simulink model "C1_Chirp_Filter"  (R2019b)
settings: Solver=VariableStepAuto  StartTime=0.0  StopTime=testtime  RelTol=1e-3
InitFcn:
  | C1_Chirp_Test_Parameters
StopFcn:
  | Verify_C1_Chirp_Filter
values from neighbouring files (symbols this model uses):
  C1gain_norm = C1gain_norm*((CF-pimag(i))^2 + (preal(i))^2)    [C1_Chirp_Test_Parameters.m]
  C1initphase = C1initphase + atan(CF/(-rzero))-atan((CF-pimag(2*i-1))/(-preal(2*i-1)))-atan((CF+pimag(2*i-1))/(-preal(2*i-1)))    [C1_Chirp_Test_Parameters.m]
  CF = 2*pi*cf    (= 6283.18530718)    [C1_Chirp_Test_Parameters.m]
  Fs = 48e3    (= 48000)    [C1_Chirp_Test_Parameters.m]
  fs_bilinear = 2*pi*cf/tan(2*pi*cf*tdres/2)    [C1_Chirp_Test_Parameters.m]
  norm_gainc1 = (sqrt(C1gain_norm))/((sqrt(CF^2+rzero^2))^order_of_zero)    [C1_Chirp_Test_Parameters.m]
  order_of_zero = half_order_pole    (= 5)    [C1_Chirp_Test_Parameters.m]
  pimag = zeros(11,1)    [C1_Chirp_Test_Parameters.m]
  preal = zeros(11,1)    [C1_Chirp_Test_Parameters.m]
  rsigma = 1    [C1_Chirp_Test_Parameters.m]
  rzero = -pzero    [C1_Chirp_Test_Parameters.m]
libraries: dspsrcs4 x2
settings Model: Creator=mblun  LastModifiedBy=t96f346
settings SFSimCC: CustomCodeUndefinedFunction=UseInterfaceOnly

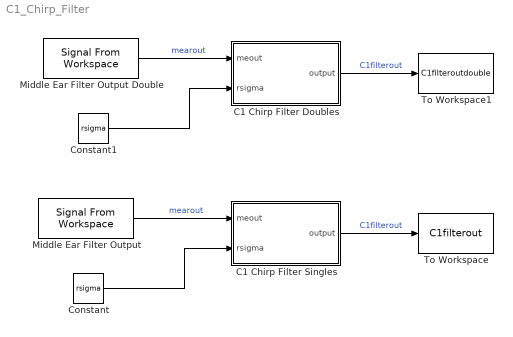
== system C1_Chirp_Filter ==
  C1 Chirp Filter Doubles : Subsystem
  C1 Chirp Filter Singles : Subsystem
  Constant : Constant  Value=rsigma  OutDataTypeStr=single  SampleTime=-1
  Constant1 : Constant  Value=rsigma  SampleTime=-1
  Middle Ear Filter Output : dspsrcs4/Signal From Workspace  X=RxSignal  Ts=1/Fs  nsamps=1  OutputAfterFinalValue=Setting to zero  ignoreOrWarnInputAndFrameLengths=off  OutputFrames=off
  Middle Ear Filter Output Double : dspsrcs4/Signal From Workspace  X=RxSignalDouble  Ts=1/Fs  nsamps=1  OutputAfterFinalValue=Setting to zero  ignoreOrWarnInputAndFrameLengths=off  OutputFrames=off
  To Workspace : ToWorkspace  VariableName=C1filterout  SampleTime=-1
      settings: Save2DSignal=2-D array (concatenate along first dimension)
  To Workspace1 : ToWorkspace  VariableName=C1filteroutdouble  SampleTime=-1
      settings: Save2DSignal=2-D array (concatenate along first dimension)
  wires:
  Middle Ear Filter Output/1 -> C1 Chirp Filter Singles/1(meout)  "mearout"
  Constant/1 -> C1 Chirp Filter Singles/2(rsigma)
  C1 Chirp Filter Singles/1(output) -> To Workspace/1  "C1filterout"
  Constant1/1 -> C1 Chirp Filter Doubles/2(rsigma)
  Middle Ear Filter Output Double/1 -> C1 Chirp Filter Doubles/1(meout)  "mearout"
  C1 Chirp Filter Doubles/1(output) -> To Workspace1/1  "C1filterout"

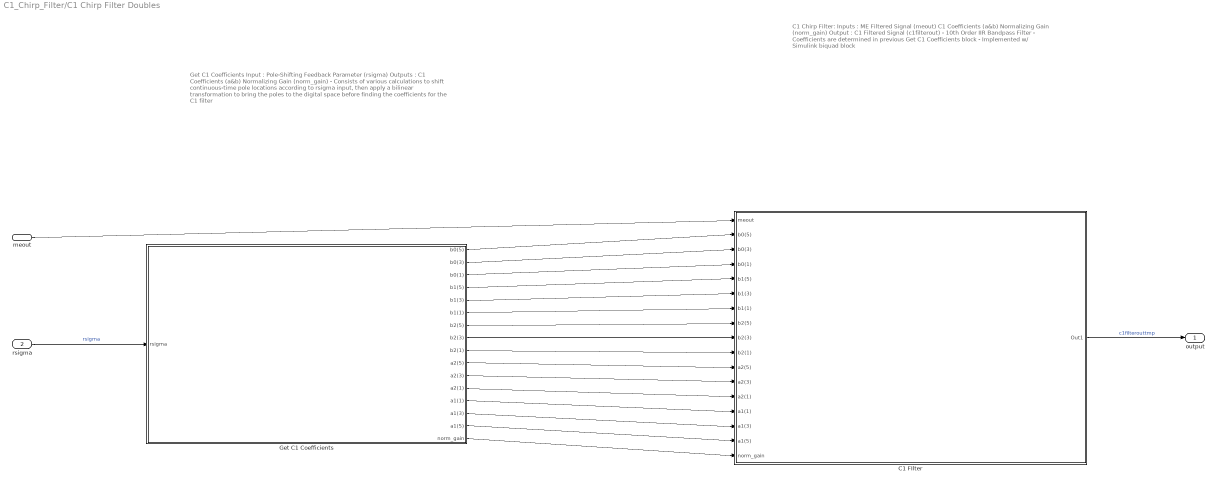
== system C1_Chirp_Filter/C1 Chirp Filter Doubles ==
  note: C1 Chirp Filter:
      |
      | Inputs : ME Filtered Signal (meout)
      | C1 Coefficients (a&b)
      | Normalizing Gain (norm_gain)
      |
      | Output : C1 Filtered Signal (c1filterout)
      |
      | - 10th Order IIR Bandpass Filter
      |
      | - Coefficients are determined in previous Get C1 Coefficients block
      |
      | - Implemented w/ Simulink biquad block
  note: Get C1 Coefficients
      |
      | Input : Pole-Shifting Feedback Parameter (rsigma)
      |
      | Outputs : C1 Coefficients (a&b)
      | Normalizing Gain (norm_gain)
      |
      | - Consists of various calculations to shift continuous-time pole locations according to rsigma input, then apply a bilinear transformation to bring the poles to the digital space before finding the coefficients for the C1 filter
  meout : Inport
  rsigma : Inport  Port=2
  C1 FIlter : Subsystem
  Get C1 Coefficients : Subsystem
  output : Outport  VectorParamsAs1DForOutWhenUnconnected=off
  wires:
  C1 FIlter/1(Out1) -> output/1  "c1filterouttmp"
  Get C1 Coefficients/1(b0(5)) -> C1 FIlter/2(b0(5))
  Get C1 Coefficients/9(b2(1)) -> C1 FIlter/10(b2(1))
  rsigma/1 -> Get C1 Coefficients/1(rsigma)  "rsigma"
  Get C1 Coefficients/10(a2(5)) -> C1 FIlter/11(a2(5))
  Get C1 Coefficients/15(a1(5)) -> C1 FIlter/16(a1(5))
  Get C1 Coefficients/6(b1(1)) -> C1 FIlter/7(b1(1))
  meout/1 -> C1 FIlter/1(meout)
  Get C1 Coefficients/16(norm_gain) -> C1 FIlter/17(norm_gain)
  Get C1 Coefficients/13(a1(1)) -> C1 FIlter/14(a1(1))
  Get C1 Coefficients/14(a1(3)) -> C1 FIlter/15(a1(3))
  Get C1 Coefficients/12(a2(1)) -> C1 FIlter/13(a2(1))
  Get C1 Coefficients/11(a2(3)) -> C1 FIlter/12(a2(3))
  Get C1 Coefficients/2(b0(3)) -> C1 FIlter/3(b0(3))
  Get C1 Coefficients/3(b0(1)) -> C1 FIlter/4(b0(1))
  Get C1 Coefficients/4(b1(5)) -> C1 FIlter/5(b1(5))
  Get C1 Coefficients/8(b2(3)) -> C1 FIlter/9(b2(3))
  Get C1 Coefficients/5(b1(3)) -> C1 FIlter/6(b1(3))
  Get C1 Coefficients/7(b2(5)) -> C1 FIlter/8(b2(5))

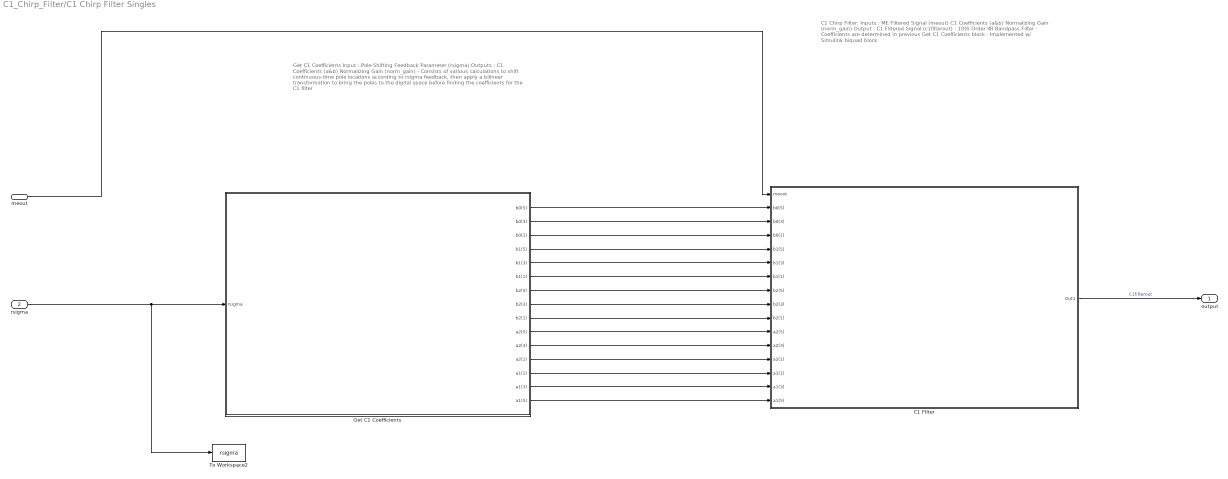
== system C1_Chirp_Filter/C1 Chirp Filter Singles ==
  note: C1 Chirp Filter:
      |
      | Inputs : ME Filtered Signal (meout)
      | C1 Coefficients (a&b)
      | Normalizing Gain (norm_gain)
      |
      | Output : C1 Filtered Signal (c1filterout)
      |
      | - 10th Order IIR Bandpass Filter
      |
      | - Coefficients are determined in previous Get C1 Coefficients block
      |
      | - Implemented w/ Simulink biquad block
  note: Get C1 Coefficients
      |
      | Input : Pole-Shifting Feedback Parameter (rsigma)
      |
      | Outputs : C1 Coefficients (a&b)
      | Normalizing Gain (norm_gain)
      |
      | - Consists of various calculations to shift continuous-time pole locations according to rsigma feedback, then apply a bilinear transformation to bring the poles to the digital space before finding the coefficients for the C1 filter
  meout : Inport
  rsigma : Inport  Port=2
  C1 FIlter : Subsystem
  Get C1 Coefficients : Subsystem
  To Workspace2 : ToWorkspace  VariableName=rsigma  SampleTime=-1
      settings: Save2DSignal=2-D array (concatenate along first dimension)
  output : Outport  VectorParamsAs1DForOutWhenUnconnected=off
  wires:
  meout/1 -> C1 FIlter/1(meout)
  Get C1 Coefficients/1(b0(5)) -> C1 FIlter/2(b0(5))
  Get C1 Coefficients/2(b0(3)) -> C1 FIlter/3(b0(3))
  Get C1 Coefficients/3(b0(1)) -> C1 FIlter/4(b0(1))
  Get C1 Coefficients/4(b1(5)) -> C1 FIlter/5(b1(5))
  Get C1 Coefficients/5(b1(3)) -> C1 FIlter/6(b1(3))
  Get C1 Coefficients/6(b1(1)) -> C1 FIlter/7(b1(1))
  Get C1 Coefficients/7(b2(5)) -> C1 FIlter/8(b2(5))
  Get C1 Coefficients/8(b2(3)) -> C1 FIlter/9(b2(3))
  Get C1 Coefficients/9(b2(1)) -> C1 FIlter/10(b2(1))
  Get C1 Coefficients/10(a2(5)) -> C1 FIlter/11(a2(5))
  Get C1 Coefficients/11(a2(3)) -> C1 FIlter/12(a2(3))
  Get C1 Coefficients/12(a2(1)) -> C1 FIlter/13(a2(1))
  Get C1 Coefficients/13(a1(1)) -> C1 FIlter/14(a1(1))
  Get C1 Coefficients/14(a1(3)) -> C1 FIlter/15(a1(3))
  Get C1 Coefficients/15(a1(5)) -> C1 FIlter/16(a1(5))
  C1 FIlter/1(Out1) -> output/1  "C1filterout"
  rsigma/1 -> To Workspace2/1, Get C1 Coefficients/1(rsigma)

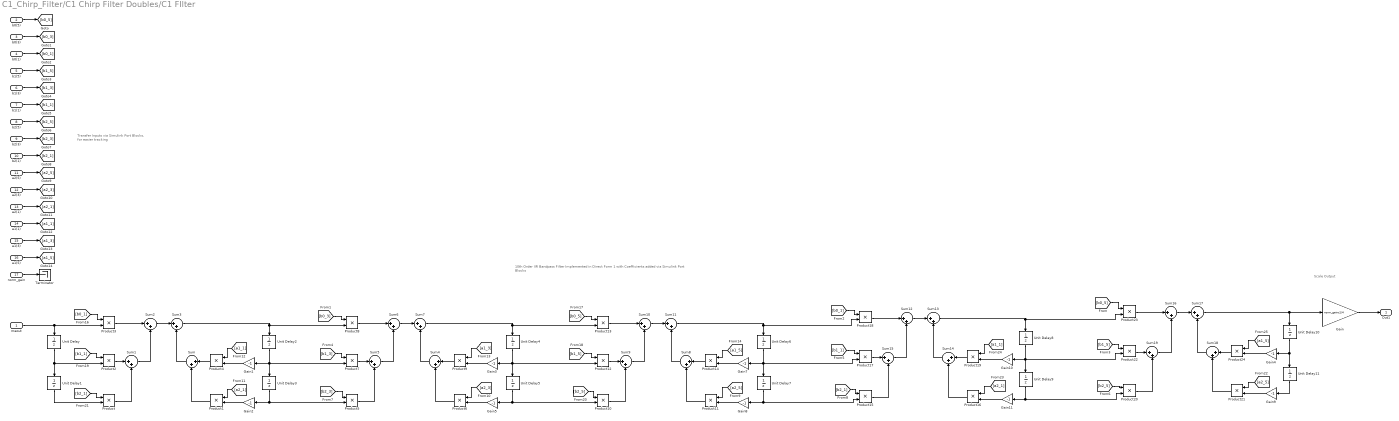
== system C1_Chirp_Filter/C1 Chirp Filter Doubles/C1 FIlter ==
  note: Transfer Inputs via Simulink Port Blocks, for easier tracking
  note: 10th Order IIR Bandpass Filter Implemented in Direct Form 1 with Coefficients added via Simulink Port Blocks
  note: Scale Output
  meout : Inport
  b0(5) : Inport  Port=2
  b0(3) : Inport  Port=3
  b0(1) : Inport  Port=4
  b1(5) : Inport  Port=5
  b1(3) : Inport  Port=6
  b1(1) : Inport  Port=7
  b2(5) : Inport  Port=8
  b2(3) : Inport  Port=9
  b2(1) : Inport  Port=10
  a2(5) : Inport  Port=11
  a2(3) : Inport  Port=12
  a2(1) : Inport  Port=13
  a1(1) : Inport  Port=14
  a1(3) : Inport  Port=15
  a1(5) : Inport  Port=16
  norm_gain : Inport  Port=17
  Gain : Gain  Gain=norm_gainc1/4
  Gain{1..5,7..11} (10 alike) : Gain  Gain=-1
  Product{,1..24} (25 alike) : Product
  Sum{,1..19} (20 alike) : Sum  Inputs=|++
  Terminator : Terminator
  Unit Delay{,1..11} (12 alike) : UnitDelay  SampleTime=-1  HasFrameUpgradeWarning=on
  Out1 : Outport  VectorParamsAs1DForOutWhenUnconnected=off
  wires:
  [a1_5] -> Product14/1
  Product15/1 -> Sum15/2
  Product16/1 -> Sum14/2
  Sum5/1 -> Sum6/2
  Sum15/1 -> Sum12/2
  Unit Delay2/1 -> Product7/2, Unit Delay3/1, Gain1/1
  Unit Delay6/1 -> Product17/2, Unit Delay7/1, Gain7/1
  [b1_3] -> Product7/1
  Sum1/1 -> Sum2/2
  [b0_1] -> Product3/1
  Product4/1 -> Sum/1
  Unit Delay8/1 -> Product22/2, Unit Delay9/1, Gain10/1
  Product12/1 -> Sum9/1
  Sum17/1 -> Unit Delay10/1, Gain/1
  Product3/1 -> Sum2/1
  [b2_3] -> Product5/1
  Sum7/1 -> Product13/2, Unit Delay4/1
  [a2_1] -> Product1/1
  [b2_1] -> Product/1
  Product24/1 -> Sum18/1
  Unit Delay3/1 -> Product5/2, Gain2/1
  Product5/1 -> Sum5/2
  Unit Delay4/1 -> Product12/2, Unit Delay5/1, Gain3/1
  Sum13/1 -> Product23/2, Unit Delay8/1
  Sum3/1 -> Product8/2, Unit Delay2/1
  Sum4/1 -> Sum7/2
  Product19/1 -> Sum14/1
  Product7/1 -> Sum5/1
  Product10/1 -> Sum9/2
  Product20/1 -> Sum19/2
  [a1_5] -> Product24/1
  Sum6/1 -> Sum7/1
  [b0_5] -> Product13/1
  [a1_3] -> Product9/1
  Product22/1 -> Sum19/1
  Product8/1 -> Sum6/1
  meout/1 -> Product3/2, Unit Delay/1
  Product2/1 -> Sum1/1
  Sum11/1 -> Product18/2, Unit Delay6/1
  Unit Delay5/1 -> Product10/2, Gain5/1
  [b1_5] -> Product12/1
  Sum2/1 -> Sum3/1
  Product11/1 -> Sum8/2
  Sum19/1 -> Sum16/2
  [b2_5] -> Product20/1
  Product14/1 -> Sum8/1
  Product18/1 -> Sum12/1
  Sum8/1 -> Sum11/2
  [b0_3] -> Product8/1
  Sum12/1 -> Sum13/1
  [b0_5] -> Product23/1
  [b0_1] -> Product18/1
  [a1_1] -> Product19/1
  [a2_5] -> Product21/1
  Unit Delay/1 -> Unit Delay1/1, Product2/2
  Product17/1 -> Sum15/1
  Unit Delay7/1 -> Product15/2, Gain8/1
  Unit Delay10/1 -> Unit Delay11/1, Gain4/1
  [a2_5] -> Product11/1
  Unit Delay11/1 -> Gain9/1
  Gain/1 -> Out1/1
  Product23/1 -> Sum16/1
  Product9/1 -> Sum4/1
  [b1_1] -> Product17/1
  Product13/1 -> Sum10/1
  Product6/1 -> Sum4/2
  Sum9/1 -> Sum10/2
  Sum16/1 -> Sum17/1
  Product21/1 -> Sum18/2
  [b1_1] -> Product2/1
  Sum18/1 -> Sum17/2
  [b1_5] -> Product22/1
  [a2_1] -> Product16/1
  [a2_3] -> Product6/1
  Sum10/1 -> Sum11/1
  [b2_5] -> Product10/1
  [b2_1] -> Product15/1
  Product/1 -> Sum1/2
  Unit Delay9/1 -> Product20/2, Gain11/1
  Sum14/1 -> Sum13/2
  [a1_1] -> Product4/1
  Sum/1 -> Sum3/2
  Unit Delay1/1 -> Product/2
  Product1/1 -> Sum/2
  b0(5)/1 -> [b0_5]
  b0(3)/1 -> [b0_3]
  b0(1)/1 -> [b0_1]
  b1(5)/1 -> [b1_5]
  b1(3)/1 -> [b1_3]
  b1(1)/1 -> [b1_1]
  b2(5)/1 -> [b2_5]
  b2(3)/1 -> [b2_3]
  b2(1)/1 -> [b2_1]
  a2(5)/1 -> [a2_5]
  a2(3)/1 -> [a2_3]
  a2(1)/1 -> [a2_1]
  a1(1)/1 -> [a1_1]
  a1(3)/1 -> [a1_3]
  a1(5)/1 -> [a1_5]
  norm_gain/1 -> Terminator/1
  Gain1/1 -> Product4/2
  Gain2/1 -> Product1/2
  Gain3/1 -> Product9/2
  Gain5/1 -> Product6/2
  Gain7/1 -> Product14/2
  Gain8/1 -> Product11/2
  Gain10/1 -> Product19/2
  Gain11/1 -> Product16/2
  Gain4/1 -> Product24/2
  Gain9/1 -> Product21/2

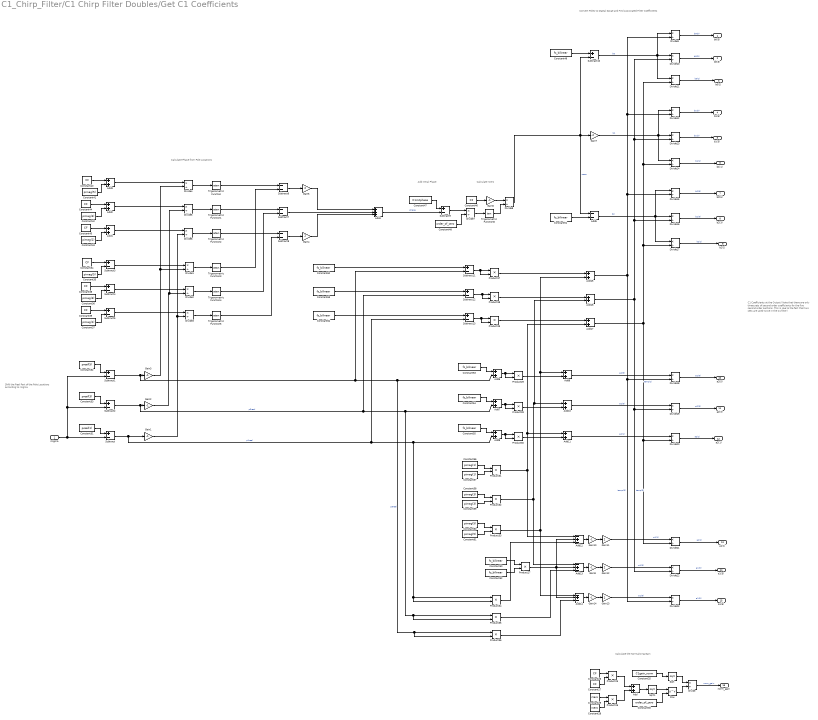
== system C1_Chirp_Filter/C1 Chirp Filter Doubles/Get C1 Coefficients ==
  note: Calculate Phase from Pole Locations
  note: Shift the Real Part of the Pole Locations according to rsigma
  note: Add Initial Phase
  note: Calculate rzero
  note: Convert Poles to Digital Spcae and Find Associated Filter Coefficients
  note: C1 Coefficients at the Output (Note that there are only three sets of second order coefficients for the five second order sections. This is due to the fact that two sets are used twice in the C1 filter)
  note: Calculate the Normalizing Gain
  rsigma : Inport
  Add{,1..3,6..11,15..17} (13 alike) : Sum
  Add12 : Sum  Inputs=-+-
  Add13 : Sum  Inputs=-+-
  Add14 : Sum  Inputs=-+-
  Add4 : Sum  Inputs=+++
  Add5 : Sum  Inputs=--
  Constant25 : Constant  Value=C1gain_norm  SampleTime=-1
  Constant{26..27,34,38..40,44..46} (9 alike) : Constant  Value=CF  SampleTime=-1
  Constant28 : Constant  Value=rzero  SampleTime=-1
  Constant29 : Constant  Value=rzero  SampleTime=-1
  Constant30 : Constant  Value=order_of_zero  SampleTime=-1
  Constant31 : Constant  Value=preal(1)  SampleTime=-1
  Constant32 : Constant  Value=preal(5)  SampleTime=-1
  Constant33 : Constant  Value=preal(3)  SampleTime=-1
  Constant{35,41,60..61} (4 alike) : Constant  Value=pimag(5)  SampleTime=-1
  Constant{36,42,58..59} (4 alike) : Constant  Value=pimag(3)  SampleTime=-1
  Constant{37,43,56..57} (4 alike) : Constant  Value=pimag(1)  SampleTime=-1
  Constant47 : Constant  Value=C1initphase  SampleTime=-1
  Constant48 : Constant  Value=order_of_zero  SampleTime=-1
  Constant{49..55,62..64} (10 alike) : Constant  Value=fs_bilinear  SampleTime=-1
  Divide{,1..23} (24 alike) : Product  Inputs=*/  SaturateOnIntegerOverflow=on  RndMeth=Zero
  Gain{1..3,6,9..10,14} (7 alike) : Gain  Gain=-1
  Gain{4..5,11..13} (5 alike) : Gain  Gain=2
  Gain7 : Gain  Gain=-2
  Pow : Math  Operator=pow  RndMeth=Zero  SaturateOnIntegerOverflow=on
  Product{25..39} (15 alike) : Product
  Sqrt : Sqrt  SaturateOnIntegerOverflow=on
  Sqrt1 : Sqrt  SaturateOnIntegerOverflow=on
  Subtract{,1..5,9..13} (11 alike) : Sum  Inputs=+-
  Subtract6 : Sum  Inputs=--
  Subtract7 : Sum  Inputs=--
  Subtract8 : Sum  Inputs=--
  Trigonometric Function{,1..5} (6 alike) : Trigonometry  Operator=atan  ApproximationMethod=CORDIC
  Trigonometric Function6 : Trigonometry  Operator=tan  ApproximationMethod=CORDIC
  b0(5) : Outport  VectorParamsAs1DForOutWhenUnconnected=off
  b0(3) : Outport  Port=2  VectorParamsAs1DForOutWhenUnconnected=off
  b0(1) : Outport  Port=3  VectorParamsAs1DForOutWhenUnconnected=off
  b1(5) : Outport  Port=4  VectorParamsAs1DForOutWhenUnconnected=off
  b1(3) : Outport  Port=5  VectorParamsAs1DForOutWhenUnconnected=off
  b1(1) : Outport  Port=6  VectorParamsAs1DForOutWhenUnconnected=off
  b2(5) : Outport  Port=7  VectorParamsAs1DForOutWhenUnconnected=off
  b2(3) : Outport  Port=8  VectorParamsAs1DForOutWhenUnconnected=off
  b2(1) : Outport  Port=9  VectorParamsAs1DForOutWhenUnconnected=off
  a2(5) : Outport  Port=10  VectorParamsAs1DForOutWhenUnconnected=off
  a2(3) : Outport  Port=11  VectorParamsAs1DForOutWhenUnconnected=off
  a2(1) : Outport  Port=12  VectorParamsAs1DForOutWhenUnconnected=off
  a1(1) : Outport  Port=13  VectorParamsAs1DForOutWhenUnconnected=off
  a1(3) : Outport  Port=14  VectorParamsAs1DForOutWhenUnconnected=off
  a1(5) : Outport  Port=15  VectorParamsAs1DForOutWhenUnconnected=off
  norm_gain : Outport  Port=16  VectorParamsAs1DForOutWhenUnconnected=off
  wires:
  Add5/1 -> Divide17/1, Divide16/1, Divide15/1  "b2"
  Constant46/1 -> Gain6/1
  Divide6/1 -> Trigonometric Function2/1
  Divide18/1 -> a2(5)/1  "a2(5)"
  Subtract9/1 -> Divide7/1
  Constant33/1 -> Subtract2/1
  Add17/1 -> Divide21/2, Divide20/2, Divide17/2, Divide11/2, Divide14/2  "temp(1)"
  Product31/1 -> Add12/1, Add17/2, Add11/1
  Gain2/1 -> Divide5/2, Divide2/2
  Subtract8/1 -> Gain4/1
  rsigma/1 -> Subtract/2, Subtract1/2, Subtract2/2
  Gain1/1 -> Divide6/2, Divide3/2
  Add12/1 -> Gain10/1
  Constant52/1 -> Product27/2
  Add13/1 -> Gain9/1
  Add15/1 -> Divide23/2, Divide18/2, Divide9/2, Divide12/2, Divide15/2  "temp(5)"
  Add14/1 -> Gain14/1
  Product27/1 -> Add14/2, Add13/2, Add12/2
  Subtract2/1 -> Subtract12/2, Product35/2, Product35/1, Add7/2, Gain2/1  "p3real"
  Subtract1/1 -> Subtract11/2, Product36/2, Product36/1, Add6/2, Gain3/1  "p5real"
  Subtract/1 -> Subtract13/2, Product34/1, Product34/2, Add8/2, Gain1/1  "p1real"
  Divide5/1 -> Trigonometric Function1/1
  Constant59/1 -> Product32/2
  Add4/1 -> Subtract9/2  "phase"
  Product30/1 -> Add11/2
  Subtract13/1 -> Product39/2, Product39/1
  Product38/1 -> Add16/1
  Product39/1 -> Add17/1
  Divide21/1 -> a1(1)/1  "a1(1)"
  Product32/1 -> Add16/2, Add10/1, Add13/1
  Subtract7/1 -> Add4/2
  Constant62/1 -> Subtract11/1
  Constant58/1 -> Product32/1
  Divide2/1 -> Trigonometric Function4/1
  Subtract10/1 -> Divide11/1, Divide10/1, Divide9/1  "b0"
  Constant31/1 -> Subtract/1
  Trigonometric Function3/1 -> Subtract6/2
  Product36/1 -> Add14/3
  Add9/1 -> Divide18/1  "a2(5)"
  Product33/1 -> Add9/1, Add15/2, Add14/1
  Constant41/1 -> Add3/2
  Constant44/1 -> Add2/1
  Gain7/1 -> Divide14/1, Divide13/1, Divide12/1  "b1"
  Product35/1 -> Add13/3
  Add16/1 -> Divide22/2, Divide19/2, Divide10/2, Divide13/2, Divide16/2  "temp(3)"
  Constant63/1 -> Subtract12/1
  Constant28/1 -> Product26/2
  Divide8/1 -> Subtract10/2, Add5/1, Gain7/1  "rzero"
  Product34/1 -> Add12/3
  Trigonometric Function4/1 -> Subtract7/2
  Trigonometric Function5/1 -> Subtract8/2
  Subtract11/1 -> Product37/2, Product37/1
  Gain11/1 -> Divide21/1  "a1(1)"
  Gain12/1 -> Divide22/1  "a1(3)"
  Constant32/1 -> Subtract1/1
  Trigonometric Function6/1 -> Divide8/2
  Divide/1 -> norm_gain/1  "norm_gain"
  Add8/1 -> Product30/2, Product30/1
  Constant40/1 -> Add3/1
  Gain6/1 -> Divide8/1
  Trigonometric Function1/1 -> Subtract7/1
  Add2/1 -> Divide5/1
  Subtract6/1 -> Gain5/1
  Gain13/1 -> Divide23/1  "a1(5)"
  Constant42/1 -> Add2/2
  Divide4/1 -> Trigonometric Function/1
  Product37/1 -> Add15/1
  Gain3/1 -> Divide4/2, Divide1/2
  Divide3/1 -> Trigonometric Function5/1
  Divide1/1 -> Trigonometric Function3/1
  Constant55/1 -> Add8/1
  Divide23/1 -> a1(5)/1  "a1(5)"
  Divide7/1 -> Trigonometric Function6/1
  Add6/1 -> Product29/2, Product29/1
  Product29/1 -> Add9/2
  Constant47/1 -> Subtract9/1
  Constant49/1 -> Subtract10/1
  Trigonometric Function2/1 -> Subtract8/1
  Subtract12/1 -> Product38/2, Product38/1
  Add3/1 -> Divide4/1
  Product25/1 -> Add/1
  Constant37/1 -> Subtract5/2
  Constant50/1 -> Product27/1
  Add11/1 -> Divide20/1  "a2(1)"
  Subtract5/1 -> Divide3/1
  Add1/1 -> Divide6/1
  Subtract4/1 -> Divide2/1
  Subtract3/1 -> Divide1/1
  Constant34/1 -> Subtract3/1
  Constant45/1 -> Add1/1
  Gain4/1 -> Add4/3
  Constant56/1 -> Product31/1
  Add7/1 -> Product28/2, Product28/1
  Constant27/1 -> Product25/2
  Gain5/1 -> Add4/1
  Constant51/1 -> Add5/2
  Product28/1 -> Add10/2
  Divide13/1 -> b1(3)/1  "b1(3)"
  Constant25/1 -> Sqrt/1
  Constant26/1 -> Product25/1
  Constant29/1 -> Product26/1
  Add/1 -> Sqrt1/1
  Sqrt/1 -> Divide/1
  Pow/1 -> Divide/2
  Sqrt1/1 -> Pow/1
  Product26/1 -> Add/2
  Constant30/1 -> Pow/2
  Constant36/1 -> Subtract4/2
  Constant39/1 -> Subtract5/1
  Constant61/1 -> Product33/2
  Constant60/1 -> Product33/1
  Constant54/1 -> Add7/1
  Constant57/1 -> Product31/2
  Constant64/1 -> Subtract13/1
  Add10/1 -> Divide19/1  "a2(3)"
  Constant38/1 -> Subtract4/1
  Trigonometric Function/1 -> Subtract6/1
  Constant35/1 -> Subtract3/2
  Constant43/1 -> Add1/2
  Constant48/1 -> Divide7/2
  Constant53/1 -> Add6/1
  Divide17/1 -> b2(1)/1  "b2(1)"
  Divide12/1 -> b1(5)/1  "b1(5)"
  Divide20/1 -> a2(1)/1  "a2(1)"
  Divide11/1 -> b0(1)/1  "b0(1)"
  Divide14/1 -> b1(1)/1  "b1(1)"
  Divide15/1 -> b2(5)/1  "b2(5)"
  Divide10/1 -> b0(3)/1  "b0(3)"
  Divide22/1 -> a1(3)/1  "a1(3)"
  Divide9/1 -> b0(5)/1  "b0(5)"
  Divide19/1 -> a2(3)/1  "a2(3)"
  Divide16/1 -> b2(3)/1  "b2(3)"
  Gain10/1 -> Gain11/1
  Gain9/1 -> Gain12/1
  Gain14/1 -> Gain13/1

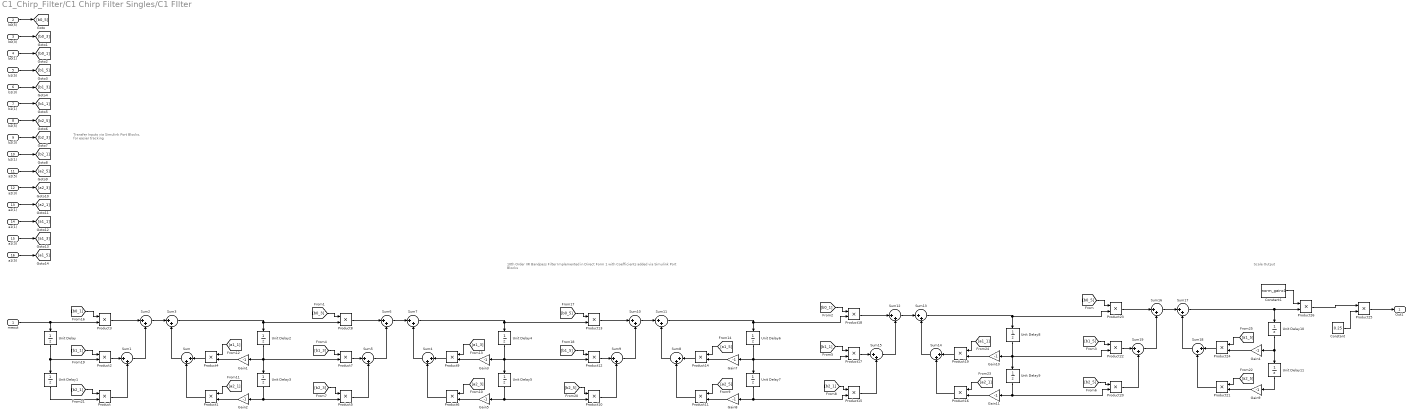
== system C1_Chirp_Filter/C1 Chirp Filter Singles/C1 FIlter ==
  note: Transfer Inputs via Simulink Port Blocks, for easier tracking
  note: 10th Order IIR Bandpass Filter Implemented in Direct Form 1 with Coefficients added via Simulink Port Blocks
  note: Scale Output
  meout : Inport  OutDataTypeStr=single
  b0(5) : Inport  Port=2  OutDataTypeStr=single
  b0(3) : Inport  Port=3  OutDataTypeStr=single
  b0(1) : Inport  Port=4  OutDataTypeStr=single
  b1(5) : Inport  Port=5  OutDataTypeStr=single
  b1(3) : Inport  Port=6  OutDataTypeStr=single
  b1(1) : Inport  Port=7  OutDataTypeStr=single
  b2(5) : Inport  Port=8  OutDataTypeStr=single
  b2(3) : Inport  Port=9  OutDataTypeStr=single
  b2(1) : Inport  Port=10  OutDataTypeStr=single
  a2(5) : Inport  Port=11  OutDataTypeStr=single
  a2(3) : Inport  Port=12  OutDataTypeStr=single
  a2(1) : Inport  Port=13  OutDataTypeStr=single
  a1(1) : Inport  Port=14  OutDataTypeStr=single
  a1(3) : Inport  Port=15  OutDataTypeStr=single
  a1(5) : Inport  Port=16  OutDataTypeStr=single
  Constant : Constant  Value=0.25  OutDataTypeStr=single  SampleTime=-1
  Constant1 : Constant  Value=norm_gainc1  OutDataTypeStr=single  SampleTime=-1
  Gain{1..5,7..11} (10 alike) : Gain  Gain=-1  OutDataTypeStr=single
  Product{,1..26} (27 alike) : Product  OutDataTypeStr=single
  Sum{,1..19} (20 alike) : Sum  Inputs=|++  OutDataTypeStr=single
  Unit Delay{,1..11} (12 alike) : UnitDelay  SampleTime=-1  HasFrameUpgradeWarning=on
  Out1 : Outport  VectorParamsAs1DForOutWhenUnconnected=off
  wires:
  [a1_5] -> Product14/1
  Product15/1 -> Sum15/2
  Product16/1 -> Sum14/2
  Sum5/1 -> Sum6/2
  Sum15/1 -> Sum12/2
  Unit Delay2/1 -> Product7/2, Unit Delay3/1, Gain1/1
  Unit Delay6/1 -> Product17/2, Unit Delay7/1, Gain7/1
  [b1_3] -> Product7/1
  Sum1/1 -> Sum2/2
  [b0_1] -> Product3/1
  Product4/1 -> Sum/1
  Unit Delay8/1 -> Product22/2, Unit Delay9/1, Gain10/1
  Product12/1 -> Sum9/1
  Sum17/1 -> Product26/2, Unit Delay10/1
  Product3/1 -> Sum2/1
  [b2_3] -> Product5/1
  Sum7/1 -> Product13/2, Unit Delay4/1
  [a2_1] -> Product1/1
  [b2_1] -> Product/1
  Product24/1 -> Sum18/1
  Unit Delay3/1 -> Product5/2, Gain2/1
  Product5/1 -> Sum5/2
  Unit Delay4/1 -> Product12/2, Unit Delay5/1, Gain3/1
  Sum13/1 -> Product23/2, Unit Delay8/1
  Sum3/1 -> Product8/2, Unit Delay2/1
  Sum4/1 -> Sum7/2
  Product19/1 -> Sum14/1
  Product7/1 -> Sum5/1
  Product10/1 -> Sum9/2
  Product20/1 -> Sum19/2
  [a1_5] -> Product24/1
  Sum6/1 -> Sum7/1
  [b0_5] -> Product13/1
  [a1_3] -> Product9/1
  Product22/1 -> Sum19/1
  Product8/1 -> Sum6/1
  meout/1 -> Product3/2, Unit Delay/1
  Product2/1 -> Sum1/1
  Sum11/1 -> Product18/2, Unit Delay6/1
  Unit Delay5/1 -> Product10/2, Gain5/1
  [b1_5] -> Product12/1
  Sum2/1 -> Sum3/1
  Product11/1 -> Sum8/2
  Sum19/1 -> Sum16/2
  [b2_5] -> Product20/1
  Product14/1 -> Sum8/1
  Product18/1 -> Sum12/1
  Sum8/1 -> Sum11/2
  [b0_3] -> Product8/1
  Sum12/1 -> Sum13/1
  [b0_5] -> Product23/1
  [b0_1] -> Product18/1
  [a1_1] -> Product19/1
  [a2_5] -> Product21/1
  Unit Delay/1 -> Unit Delay1/1, Product2/2
  Product17/1 -> Sum15/1
  Unit Delay7/1 -> Product15/2, Gain8/1
  Unit Delay10/1 -> Unit Delay11/1, Gain4/1
  [a2_5] -> Product11/1
  Unit Delay11/1 -> Gain9/1
  Product25/1 -> Out1/1
  Product23/1 -> Sum16/1
  Product9/1 -> Sum4/1
  [b1_1] -> Product17/1
  Product13/1 -> Sum10/1
  Product6/1 -> Sum4/2
  Sum9/1 -> Sum10/2
  Sum16/1 -> Sum17/1
  Product21/1 -> Sum18/2
  [b1_1] -> Product2/1
  Sum18/1 -> Sum17/2
  [b1_5] -> Product22/1
  [a2_1] -> Product16/1
  [a2_3] -> Product6/1
  Sum10/1 -> Sum11/1
  [b2_5] -> Product10/1
  [b2_1] -> Product15/1
  Product/1 -> Sum1/2
  Unit Delay9/1 -> Product20/2, Gain11/1
  Sum14/1 -> Sum13/2
  [a1_1] -> Product4/1
  Sum/1 -> Sum3/2
  Unit Delay1/1 -> Product/2
  Product1/1 -> Sum/2
  b0(5)/1 -> [b0_5]
  b0(3)/1 -> [b0_3]
  b0(1)/1 -> [b0_1]
  b1(5)/1 -> [b1_5]
  b1(3)/1 -> [b1_3]
  b1(1)/1 -> [b1_1]
  b2(5)/1 -> [b2_5]
  b2(3)/1 -> [b2_3]
  b2(1)/1 -> [b2_1]
  a2(5)/1 -> [a2_5]
  a2(3)/1 -> [a2_3]
  a2(1)/1 -> [a2_1]
  a1(1)/1 -> [a1_1]
  a1(3)/1 -> [a1_3]
  a1(5)/1 -> [a1_5]
  Gain1/1 -> Product4/2
  Gain2/1 -> Product1/2
  Gain3/1 -> Product9/2
  Gain5/1 -> Product6/2
  Gain7/1 -> Product14/2
  Gain8/1 -> Product11/2
  Gain10/1 -> Product19/2
  Gain11/1 -> Product16/2
  Gain4/1 -> Product24/2
  Gain9/1 -> Product21/2
  Constant/1 -> Product25/2
  Product26/1 -> Product25/1
  Constant1/1 -> Product26/1

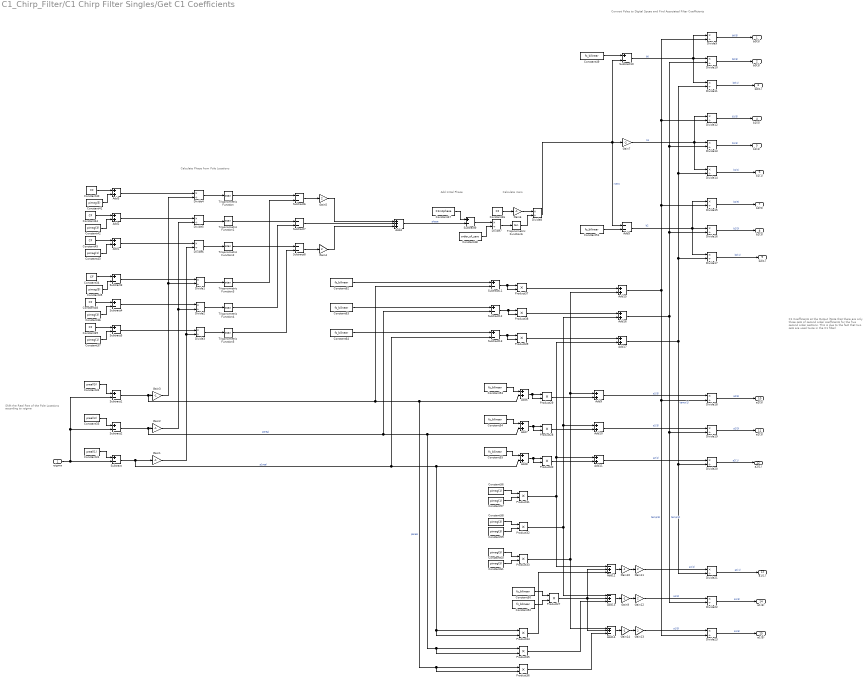
== system C1_Chirp_Filter/C1 Chirp Filter Singles/Get C1 Coefficients ==
  note: Calculate Phase from Pole Locations
  note: Shift the Real Part of the Pole Locations according to rsigma
  note: Add Initial Phase
  note: Calculate rzero
  note: Convert Poles to Digital Spcae and Find Associated Filter Coefficients
  note: C1 Coefficients at the Output (Note that there are only three sets of second order coefficients for the five second order sections. This is due to the fact that two sets are used twice in the C1 filter)
  rsigma : Inport  OutDataTypeStr=single
  Add{1..3,6..11,15..17} (12 alike) : Sum
  Add12 : Sum  Inputs=-+-
  Add13 : Sum  Inputs=-+-
  Add14 : Sum  Inputs=-+-
  Add4 : Sum  Inputs=+++
  Add5 : Sum  Inputs=--
  Constant31 : Constant  Value=preal(1)  OutDataTypeStr=single  SampleTime=-1
  Constant32 : Constant  Value=preal(5)  OutDataTypeStr=single  SampleTime=-1
  Constant33 : Constant  Value=preal(3)  OutDataTypeStr=single  SampleTime=-1
  Constant{34,38..40,44..46} (7 alike) : Constant  Value=CF  OutDataTypeStr=single  SampleTime=-1
  Constant{35,41,60..61} (4 alike) : Constant  Value=pimag(5)  OutDataTypeStr=single  SampleTime=-1
  Constant{36,42,58..59} (4 alike) : Constant  Value=pimag(3)  OutDataTypeStr=single  SampleTime=-1
  Constant{37,43,56..57} (4 alike) : Constant  Value=pimag(1)  OutDataTypeStr=single  SampleTime=-1
  Constant47 : Constant  Value=C1initphase  OutDataTypeStr=single  SampleTime=-1
  Constant48 : Constant  Value=order_of_zero  OutDataTypeStr=single  SampleTime=-1
  Constant{49..55,62..64} (10 alike) : Constant  Value=fs_bilinear  OutDataTypeStr=single  SampleTime=-1
  Divide{1..23} (23 alike) : Product  Inputs=*/  SaturateOnIntegerOverflow=on  RndMeth=Zero
  Gain{1..3,6,9..10,14} (7 alike) : Gain  Gain=-1
  Gain{4..5,11..13} (5 alike) : Gain  Gain=2
  Gain7 : Gain  Gain=-2
  Product{27..39} (13 alike) : Product
  Subtract{,1..5,9..13} (11 alike) : Sum  Inputs=+-
  Subtract6 : Sum  Inputs=--
  Subtract7 : Sum  Inputs=--
  Subtract8 : Sum  Inputs=--
  Trigonometric Function{,1..5} (6 alike) : Trigonometry  Operator=atan  ApproximationMethod=CORDIC
  Trigonometric Function6 : Trigonometry  Operator=tan  ApproximationMethod=CORDIC
  b0(5) : Outport  OutDataTypeStr=single  VectorParamsAs1DForOutWhenUnconnected=off
  b0(3) : Outport  Port=2  OutDataTypeStr=single  VectorParamsAs1DForOutWhenUnconnected=off
  b0(1) : Outport  Port=3  OutDataTypeStr=single  VectorParamsAs1DForOutWhenUnconnected=off
  b1(5) : Outport  Port=4  OutDataTypeStr=single  VectorParamsAs1DForOutWhenUnconnected=off
  b1(3) : Outport  Port=5  OutDataTypeStr=single  VectorParamsAs1DForOutWhenUnconnected=off
  b1(1) : Outport  Port=6  OutDataTypeStr=single  VectorParamsAs1DForOutWhenUnconnected=off
  b2(5) : Outport  Port=7  OutDataTypeStr=single  VectorParamsAs1DForOutWhenUnconnected=off
  b2(3) : Outport  Port=8  OutDataTypeStr=single  VectorParamsAs1DForOutWhenUnconnected=off
  b2(1) : Outport  Port=9  OutDataTypeStr=single  VectorParamsAs1DForOutWhenUnconnected=off
  a2(5) : Outport  Port=10  OutDataTypeStr=single  VectorParamsAs1DForOutWhenUnconnected=off
  a2(3) : Outport  Port=11  OutDataTypeStr=single  VectorParamsAs1DForOutWhenUnconnected=off
  a2(1) : Outport  Port=12  OutDataTypeStr=single  VectorParamsAs1DForOutWhenUnconnected=off
  a1(1) : Outport  Port=13  OutDataTypeStr=single  VectorParamsAs1DForOutWhenUnconnected=off
  a1(3) : Outport  Port=14  OutDataTypeStr=single  VectorParamsAs1DForOutWhenUnconnected=off
  a1(5) : Outport  Port=15  OutDataTypeStr=single  VectorParamsAs1DForOutWhenUnconnected=off
  wires:
  Add5/1 -> Divide17/1, Divide16/1, Divide15/1  "b2"
  Constant46/1 -> Gain6/1
  Divide6/1 -> Trigonometric Function2/1
  Divide18/1 -> a2(5)/1  "a2(5)"
  Subtract9/1 -> Divide7/1
  Constant33/1 -> Subtract2/1
  Add17/1 -> Divide21/2, Divide20/2, Divide17/2, Divide11/2, Divide14/2  "temp(1)"
  Product31/1 -> Add12/1, Add17/2, Add11/1
  Gain2/1 -> Divide5/2, Divide2/2
  Subtract8/1 -> Gain4/1
  rsigma/1 -> Subtract/2, Subtract1/2, Subtract2/2
  Gain1/1 -> Divide6/2, Divide3/2
  Add12/1 -> Gain10/1
  Constant52/1 -> Product27/2
  Add13/1 -> Gain9/1
  Add15/1 -> Divide23/2, Divide18/2, Divide9/2, Divide12/2, Divide15/2  "temp(5)"
  Add14/1 -> Gain14/1
  Product27/1 -> Add14/2, Add13/2, Add12/2
  Subtract2/1 -> Subtract12/2, Product35/2, Product35/1, Add7/2, Gain2/1  "p3real"
  Subtract1/1 -> Subtract11/2, Product36/2, Product36/1, Add6/2, Gain3/1  "p5real"
  Subtract/1 -> Subtract13/2, Product34/1, Product34/2, Add8/2, Gain1/1  "p1real"
  Divide5/1 -> Trigonometric Function1/1
  Constant59/1 -> Product32/2
  Add4/1 -> Subtract9/2  "phase"
  Product30/1 -> Add11/2
  Subtract13/1 -> Product39/2, Product39/1
  Product38/1 -> Add16/1
  Product39/1 -> Add17/1
  Divide21/1 -> a1(1)/1  "a1(1)"
  Product32/1 -> Add16/2, Add10/1, Add13/1
  Subtract7/1 -> Add4/2
  Constant62/1 -> Subtract11/1
  Constant58/1 -> Product32/1
  Divide2/1 -> Trigonometric Function4/1
  Subtract10/1 -> Divide11/1, Divide10/1, Divide9/1  "b0"
  Constant31/1 -> Subtract/1
  Trigonometric Function3/1 -> Subtract6/2
  Product36/1 -> Add14/3
  Add9/1 -> Divide18/1  "a2(5)"
  Product33/1 -> Add9/1, Add15/2, Add14/1
  Constant41/1 -> Add3/2
  Constant44/1 -> Add2/1
  Gain7/1 -> Divide14/1, Divide13/1, Divide12/1  "b1"
  Product35/1 -> Add13/3
  Add16/1 -> Divide22/2, Divide19/2, Divide10/2, Divide13/2, Divide16/2  "temp(3)"
  Constant63/1 -> Subtract12/1
  Divide8/1 -> Subtract10/2, Add5/1, Gain7/1  "rzero"
  Product34/1 -> Add12/3
  Trigonometric Function4/1 -> Subtract7/2
  Trigonometric Function5/1 -> Subtract8/2
  Subtract11/1 -> Product37/2, Product37/1
  Gain11/1 -> Divide21/1  "a1(1)"
  Gain12/1 -> Divide22/1  "a1(3)"
  Constant32/1 -> Subtract1/1
  Trigonometric Function6/1 -> Divide8/2
  Add8/1 -> Product30/2, Product30/1
  Constant40/1 -> Add3/1
  Gain6/1 -> Divide8/1
  Trigonometric Function1/1 -> Subtract7/1
  Add2/1 -> Divide5/1
  Subtract6/1 -> Gain5/1
  Gain13/1 -> Divide23/1  "a1(5)"
  Constant42/1 -> Add2/2
  Divide4/1 -> Trigonometric Function/1
  Product37/1 -> Add15/1
  Gain3/1 -> Divide4/2, Divide1/2
  Divide3/1 -> Trigonometric Function5/1
  Divide1/1 -> Trigonometric Function3/1
  Constant55/1 -> Add8/1
  Divide23/1 -> a1(5)/1  "a1(5)"
  Divide7/1 -> Trigonometric Function6/1
  Add6/1 -> Product29/2, Product29/1
  Product29/1 -> Add9/2
  Constant47/1 -> Subtract9/1
  Constant49/1 -> Subtract10/1
  Trigonometric Function2/1 -> Subtract8/1
  Subtract12/1 -> Product38/2, Product38/1
  Add3/1 -> Divide4/1
  Constant37/1 -> Subtract5/2
  Constant50/1 -> Product27/1
  Add11/1 -> Divide20/1  "a2(1)"
  Subtract5/1 -> Divide3/1
  Add1/1 -> Divide6/1
  Subtract4/1 -> Divide2/1
  Subtract3/1 -> Divide1/1
  Constant34/1 -> Subtract3/1
  Constant45/1 -> Add1/1
  Gain4/1 -> Add4/3
  Constant56/1 -> Product31/1
  Add7/1 -> Product28/2, Product28/1
  Gain5/1 -> Add4/1
  Constant51/1 -> Add5/2
  Product28/1 -> Add10/2
  Divide13/1 -> b1(3)/1  "b1(3)"
  Constant36/1 -> Subtract4/2
  Constant39/1 -> Subtract5/1
  Constant61/1 -> Product33/2
  Constant60/1 -> Product33/1
  Constant54/1 -> Add7/1
  Constant57/1 -> Product31/2
  Constant64/1 -> Subtract13/1
  Add10/1 -> Divide19/1  "a2(3)"
  Constant38/1 -> Subtract4/1
  Trigonometric Function/1 -> Subtract6/1
  Constant35/1 -> Subtract3/2
  Constant43/1 -> Add1/2
  Constant48/1 -> Divide7/2
  Constant53/1 -> Add6/1
  Divide17/1 -> b2(1)/1  "b2(1)"
  Divide12/1 -> b1(5)/1  "b1(5)"
  Divide20/1 -> a2(1)/1  "a2(1)"
  Divide11/1 -> b0(1)/1  "b0(1)"
  Divide14/1 -> b1(1)/1  "b1(1)"
  Divide15/1 -> b2(5)/1  "b2(5)"
  Divide10/1 -> b0(3)/1  "b0(3)"
  Divide22/1 -> a1(3)/1  "a1(3)"
  Divide9/1 -> b0(5)/1  "b0(5)"
  Divide19/1 -> a2(3)/1  "a2(3)"
  Divide16/1 -> b2(3)/1  "b2(3)"
  Gain10/1 -> Gain11/1
  Gain9/1 -> Gain12/1
  Gain14/1 -> Gain13/1
